simulink model "n02_NonlinearModel"  (R2021a)
settings: Solver=VariableStepAuto  StartTime=0.0  StopTime=10.0  RelTol=1e-3
values from neighbouring files (symbols this model uses):
  K_bb = g * m_b * r_arm * r_b^2 / (L_beam * (m_b*r_b^2 + J_b))    (= 0.04178613396)    [SystemModels.m]    (also in n01_UncertainSystemModels.m = 0.418287728723; n02_NonlinearModel.m = 0.0418287728723)
libraries: RCTblocks x3, cstblocks x1
settings Model: Creator=MarcosRPesanteColón  LastModifiedBy=MarcosRPesanteColón

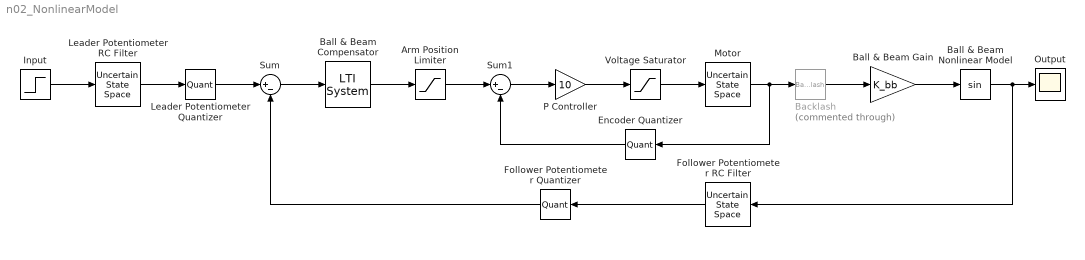
== system n02_NonlinearModel ==
  Arm Position Limiter : Saturate  UpperLimit=pi/2  LowerLimit=-pi/2
  Backlash : Backlash  Commented=through  BacklashWidth=0.25*pi/180
  Ball & Beam Compensator : cstblocks/LTI System  sys=G_c  IC=[]
  Ball & Beam Gain : Gain  Gain=K_bb
  Ball & Beam Nonlinear Model : Trigonometry  OutputSignalType=real
  Encoder Quantizer : Quantizer  QuantizationInterval=pi/2048
  Follower Potentiometer Quantizer : Quantizer  QuantizationInterval=0.4255/4096
  Follower Potentiometer RC Filter : RCTblocks/Uncertain State Space  Tag=USS  USystem=G_f  UValue=[]  X0=[]  uX0=[]
      settings: SourceProductBaseCode=RC
  Input : Step  SampleTime=0
  Leader Potentiometer Quantizer : Quantizer  QuantizationInterval=0.4255/4096
  Leader Potentiometer RC Filter : RCTblocks/Uncertain State Space  Tag=USS  USystem=G_f  UValue=[]  X0=[]  uX0=[]
      settings: SourceProductBaseCode=RC
  Motor : RCTblocks/Uncertain State Space  Tag=USS  USystem=G_m  UValue=[]  X0=[]  uX0=[]
      settings: SourceProductBaseCode=RC
  Output : Scope
  P Controller : Gain  Gain=10
  Sum : Sum  Inputs=|+-
  Sum1 : Sum  Inputs=|+-
  Voltage Saturator : Saturate  UpperLimit=5  LowerLimit=-5
  wires:
  Sum1/1 -> P Controller/1
  P Controller/1 -> Voltage Saturator/1
  Sum/1 -> Ball & Beam Compensator/1
  Ball & Beam Nonlinear Model/1 -> Follower Potentiometer RC Filter/1, Output/1
  Voltage Saturator/1 -> Motor/1
  Encoder Quantizer/1 -> Sum1/2
  Follower Potentiometer Quantizer/1 -> Sum/2
  Motor/1 -> Backlash/1, Encoder Quantizer/1
  Ball & Beam Compensator/1 -> Arm Position Limiter/1
  Arm Position Limiter/1 -> Sum1/1
  Leader Potentiometer Quantizer/1 -> Sum/1
  Follower Potentiometer RC Filter/1 -> Follower Potentiometer Quantizer/1
  Input/1 -> Leader Potentiometer RC Filter/1
  Leader Potentiometer RC Filter/1 -> Leader Potentiometer Quantizer/1
  Backlash/1 -> Ball & Beam Gain/1
  Ball & Beam Gain/1 -> Ball & Beam Nonlinear Model/1
